simulink model "model_fuzzy"  (R2022b)
settings: Solver=VariableStepAuto  StartTime=0.0  StopTime=1000  MinStep=1e-6  RelTol=1e-4
values from neighbouring files (symbols this model uses):
  atau_D = alpha*tau_D    (= 0.455)    [FIS_script.m]    (also in PID_paramaters.m)
  tau_D = 3.64    [FIS_script.m]    (also in PID_paramaters.m)
libraries: fuzblock x2, slpidlib x1
settings Model: Creator=thapl  LastModifiedBy=thapl
settings DataIOCC: SaveFormat=Array

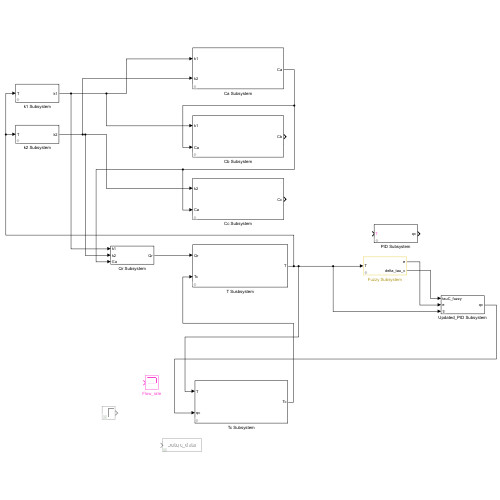
[thumbnail: Simulink's stored preview of the top-level diagram]
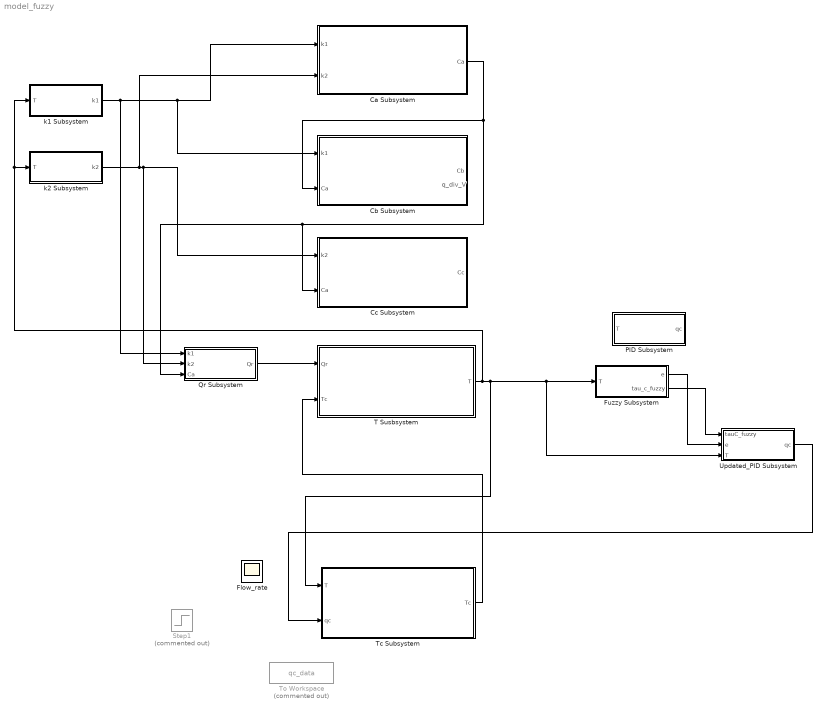
== system model_fuzzy ==
  note: q_div_V
  Ca Subsystem : Subsystem  mask{q=0.015, V=0.23, Caf=4.22}
      mask prompts: q "Feed flow rate(q)"; V "Reactor Volume(V)"; Caf "Feed Conc (Caf)"
  Cb Subsystem : Subsystem  mask{q=0.015, V=0.23, Cbf=0}
      mask prompts: q "Feed flow rate(q)"; V "Reactor Volume(V)"; Cbf "Feed Conc (Cbf)"
  Cc Subsystem : Subsystem  mask{q=0.015, V=0.23, Ccf=0}
      mask prompts: q "Feed flow rate(q)"; V "Reactor Volume(V)"; Ccf "Feed Conc (Ccf)"
  Flow_rate : Scope
  Fuzzy Subsystem : Subsystem  mask{Tset=315}
      mask prompts: Tset "Setpoint Tempreture"
  PID Subsystem : Subsystem  mask{Tset=315}
      mask prompts: Tset "Setpoint Tempreture"
  Qr Subsystem : Subsystem  mask{V=0.23, dH1=-8.6e4, dH2=-1.82e4}
      mask prompts: V "Reactor Volume (V)"; dH1 "Enthapy of Rxn1 (dH1)"; dH2 "Enthalpy of Rxn2 (dH2)"
  Step1 : Step  Commented=on  Time=200  Before=0.005  After=0.010  SampleTime=0
  T Susbsystem : Subsystem  mask{q=0.015, V=0.23, Tf=311, A=1.51, u=42.8, rho=1020, Cp=4.02}
      mask prompts: q "Reactor Flow rate (q)"; V "Reactor Volume (V)"; Tf "Inlet Fluid Temp (Tf)"; A "Contact Area (A)"; u "HTC (u)"; rho "Fluid Density (rho)"; Cp "Specific Heat capactiy (Cp)"
  Tc Subsystem : Subsystem  mask{Vc=0.21, Tcf=292, A=1.51, u=42.8, Cpc=4.182, rhoc=998}
      mask prompts: Vc "Jacket Volume (Vc)"; Tcf "Inlet Cooling Fluid Tempreture (Tcf)"; A "Contact Area (A)"; u "HTC"; Cpc "Specidic Heat Capacity of cooling fluid (Cpc)"; rhoc "Cooling Fluid Density (rhoc)"
  To Workspace : ToWorkspace  Commented=on  VariableName=qc_data  SampleTime=-1
  Updated_PID Subsystem : Subsystem  mask{t0=7.27, Kp=-480.505, tauP=27.27}
      mask prompts: t0 "Dead time"; Kp "Process Gain"; tauP "Time constant"
  k1 Subsystem : Subsystem  mask{R=8.314, k10=1.55e11, Ea1=9850*8.314}
      mask prompts: R "Universal Gas Constant(R)"; k10 "Pre exponential factor(k10)"; Ea1 "Actvation Energy(Ea1)"
  k2 Subsystem : Subsystem  mask{R=8.314, k20=4.55e25, Ea2=22019*8.314}
      mask prompts: R "Universal Gas Constant(R)"; k20 "Pre exponential factor(k10)"; Ea2 "Actvation Energy(Ea1)"
  wires:
  k1 Subsystem/1(k1) -> Ca Subsystem/1(k1), Cb Subsystem/1(k1), Qr Subsystem/1(k1)
  k2 Subsystem/1(k2) -> Qr Subsystem/2(k2), Cc Subsystem/1(k2), Ca Subsystem/2(k2)
  Ca Subsystem/1(Ca) -> Qr Subsystem/3(Ca), Cc Subsystem/2(Ca), Cb Subsystem/2(Ca)
  Tc Subsystem/1(Tc) -> T Susbsystem/2(Tc)
  T Susbsystem/1(T) -> k2 Subsystem/1(T), k1 Subsystem/1(T), Updated_PID Subsystem/3(T), Fuzzy Subsystem/1(T), Tc Subsystem/1(T)
  Qr Subsystem/1(Qr) -> T Susbsystem/1(Qr)
  Fuzzy Subsystem/1(e) -> Updated_PID Subsystem/2(e)
  Updated_PID Subsystem/1(qc) -> Tc Subsystem/2(qc)
  Fuzzy Subsystem/2(tau_c_fuzzy) -> Updated_PID Subsystem/1(tauC_fuzzy)

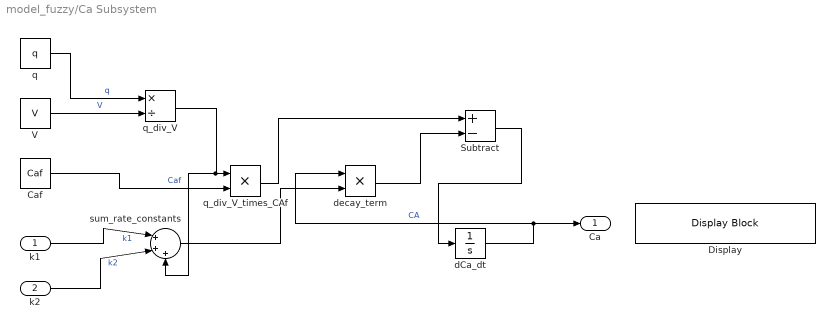
== system model_fuzzy/Ca Subsystem ==
  k1 : Inport
  k2 : Inport  Port=2
  Caf : Constant  Value=Caf
  Display : DisplayBlock  LabelPosition=Hide  Transparency=1
  Subtract : Sum  Inputs=+-
  V : Constant  Value=V
  dCa_dt : Integrator  InitialCondition=4.22
  decay_term : Product
  q : Constant  Value=q
  q_div_V : Product  Inputs=*/
  q_div_V_times_CAf : Product
  sum_rate_constants : Sum  Inputs=|+++
  Ca : Outport
  wires:
  q/1 -> q_div_V/1  "q"
  V/1 -> q_div_V/2  "V"
  q_div_V/1 -> sum_rate_constants/3, q_div_V_times_CAf/1
  Caf/1 -> q_div_V_times_CAf/2  "Caf"
  k1/1 -> sum_rate_constants/1  "k1"
  k2/1 -> sum_rate_constants/2  "k2"
  sum_rate_constants/1 -> decay_term/2
  dCa_dt/1 -> decay_term/1, Ca/1  "CA"
  decay_term/1 -> Subtract/2
  Subtract/1 -> dCa_dt/1
  q_div_V_times_CAf/1 -> Subtract/1

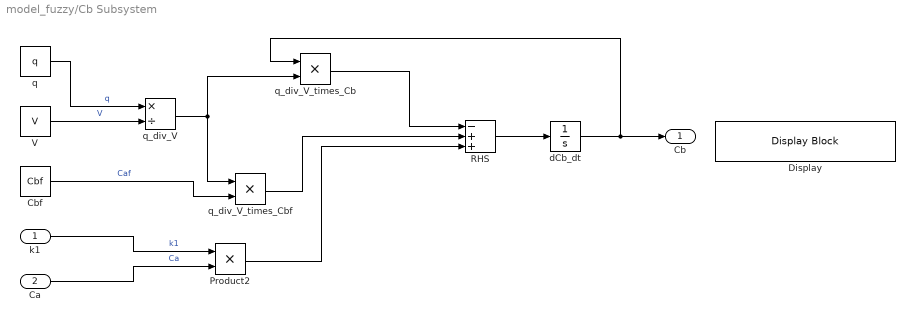
== system model_fuzzy/Cb Subsystem ==
  k1 : Inport
  Ca : Inport  Port=2
  Cbf : Constant  Value=Cbf
  Display : DisplayBlock  LabelPosition=Hide  Transparency=1
  Product2 : Product
  RHS : Sum  Inputs=-++
  V : Constant  Value=V
  dCb_dt : Integrator
  q : Constant  Value=q
  q_div_V : Product  Inputs=*/
  q_div_V_times_Cb : Product
  q_div_V_times_Cbf : Product
  Cb : Outport
  wires:
  q/1 -> q_div_V/1  "q"
  V/1 -> q_div_V/2  "V"
  q_div_V/1 -> q_div_V_times_Cb/2, q_div_V_times_Cbf/1
  Cbf/1 -> q_div_V_times_Cbf/2  "Caf"
  k1/1 -> Product2/1  "k1"
  dCb_dt/1 -> Cb/1, q_div_V_times_Cb/1
  RHS/1 -> dCb_dt/1
  Ca/1 -> Product2/2  "Ca"
  q_div_V_times_Cb/1 -> RHS/1
  q_div_V_times_Cbf/1 -> RHS/2
  Product2/1 -> RHS/3

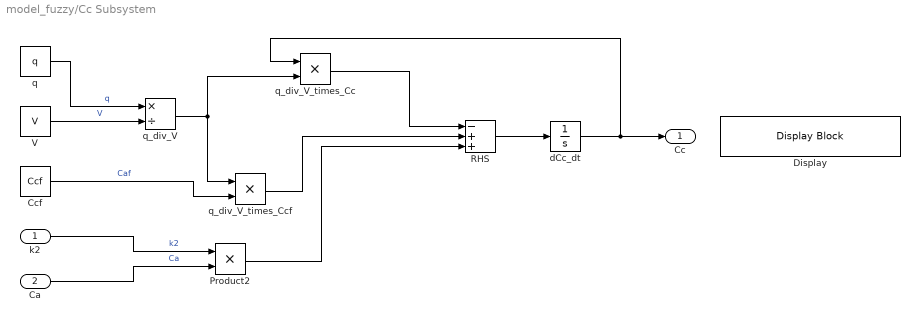
== system model_fuzzy/Cc Subsystem ==
  k2 : Inport
  Ca : Inport  Port=2
  Ccf : Constant  Value=Ccf
  Display : DisplayBlock  LabelPosition=Hide  Transparency=1
  Product2 : Product
  RHS : Sum  Inputs=-++
  V : Constant  Value=V
  dCc_dt : Integrator
  q : Constant  Value=q
  q_div_V : Product  Inputs=*/
  q_div_V_times_Cc : Product
  q_div_V_times_Ccf : Product
  Cc : Outport
  wires:
  q/1 -> q_div_V/1  "q"
  V/1 -> q_div_V/2  "V"
  q_div_V/1 -> q_div_V_times_Cc/2, q_div_V_times_Ccf/1
  Ccf/1 -> q_div_V_times_Ccf/2  "Caf"
  k2/1 -> Product2/1  "k2"
  dCc_dt/1 -> Cc/1, q_div_V_times_Cc/1
  RHS/1 -> dCc_dt/1
  Ca/1 -> Product2/2  "Ca"
  q_div_V_times_Cc/1 -> RHS/1
  q_div_V_times_Ccf/1 -> RHS/2
  Product2/1 -> RHS/3

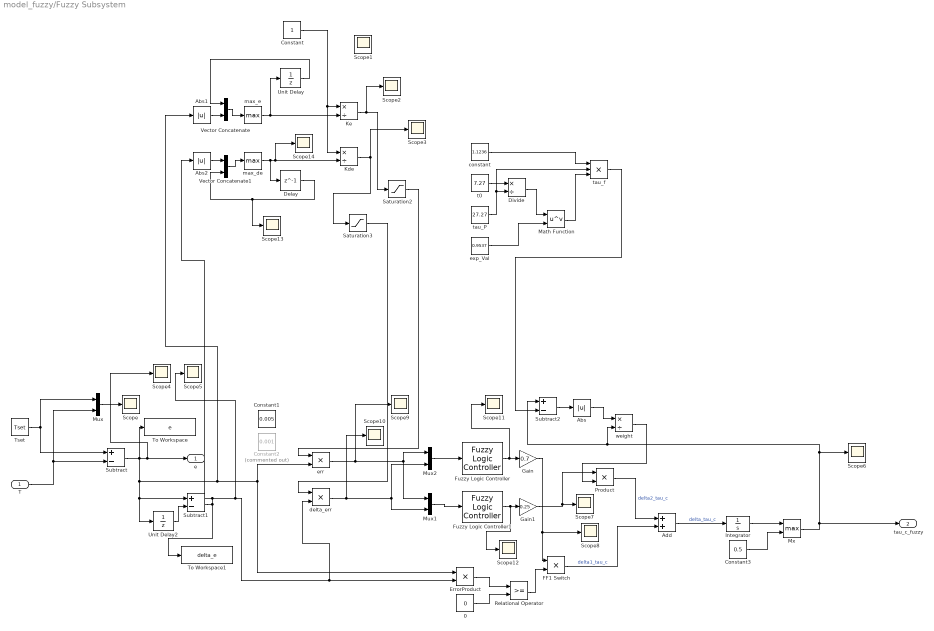
== system model_fuzzy/Fuzzy Subsystem ==
  T : Inport
  0 : Constant  Value=0
  Abs : Abs  SaturateOnIntegerOverflow=off
  Abs1 : Abs  SaturateOnIntegerOverflow=off
  Abs2 : Abs  SaturateOnIntegerOverflow=off
  Add : Sum
  Constant : Constant
  Constant1 : Constant  Value=0.005
  Constant2 : Constant  Commented=on  Value=0.001
  Constant3 : Constant  Value=0.5
  Delay : Delay  DelayLength=1  InitialCondition=0
  Divide : Product  Inputs=*/
  ErrorProduct : Product
  FF1 Switch : Product
  Fuzzy Logic Controller : fuzblock/Fuzzy Logic  Controller  FIS='FF1'  OutputSampleNumber=101  DataType=double  FuzzifiedInputs=off  RuleFiringStrengths=off  RuleOutputs=off  AggregatedOutputs=off  SimulateUsing=Interpreted execution  OutOfRangeInputValueMessage=warning  NoRuleFiredMessage=warning  EmptyOutputFuzzySetMessage=warning
  Fuzzy Logic Controller1 : fuzblock/Fuzzy Logic  Controller  FIS='FF2'  OutputSampleNumber=101  DataType=double  FuzzifiedInputs=off  RuleFiringStrengths=off  RuleOutputs=off  AggregatedOutputs=off  SimulateUsing=Interpreted execution  OutOfRangeInputValueMessage=warning  NoRuleFiredMessage=warning  EmptyOutputFuzzySetMessage=warning
  Gain : Gain  Gain=0.7
  Gain1 : Gain  Gain=0.25
  Integrator : Integrator  InitialCondition=8.6842
  Kde : Product  Inputs=*/
  Ke : Product  Inputs=*/
  Math Function : Math  Operator=pow
  Mux : Mux  Inputs=2
  Mux1 : Mux  Inputs=2
  Mux2 : Mux  Inputs=2
  Mx : MinMax  Function=max  Inputs=2
  Product : Product
  Relational Operator : RelationalOperator  OutDataTypeStr=boolean  RndMeth=Simplest  InputSameDT=off
  Saturation2 : Saturate  UpperLimit=1  LowerLimit=0.01
  Saturation3 : Saturate  UpperLimit=1  LowerLimit=0.01
  Scope{,1..14} (15 alike) : Scope
  Subtract : Sum  Inputs=+-
  Subtract1 : Sum  Inputs=+-
  Subtract2 : Sum  Inputs=+-
  To Workspace : ToWorkspace  VariableName=e  SampleTime=-1
  To Workspace1 : ToWorkspace  VariableName=delta_e  SampleTime=-1
  Tset : Constant  Value=Tset  VectorParams1D=off
  Unit Delay : UnitDelay  InitialCondition=0.1  SampleTime=-1  HasFrameUpgradeWarning=on
  Unit Delay2 : UnitDelay  InitialCondition=4  SampleTime=-1  HasFrameUpgradeWarning=on
  Vector Concatenate : Concatenate
  Vector Concatenate1 : Concatenate
  constant : Constant  Value=1.1236
  delta_err : Product
  err : Product
  exp_Val : Constant  Value=0.9537
  max_de : MinMax  Function=max
  max_e : MinMax  Function=max
  t0 : Constant  Value=7.27
  tau_P : Constant  Value=27.27
  tau_f : Product  Inputs=3
  weight : Product  Inputs=*/
  e : Outport
  tau_c_fuzzy : Outport  Port=2
  wires:
  Tset/1 -> Subtract/1, Mux/1
  Mux/1 -> Scope/1
  T/1 -> Mux/2, Subtract/2
  Unit Delay2/1 -> Subtract1/2
  Subtract2/1 -> Abs/1
  Relational Operator/1 -> FF1 Switch/2
  Subtract1/1 -> Abs2/1, Scope5/1, delta_err/2, ErrorProduct/2, To Workspace1/1
  Subtract/1 -> Unit Delay2/1, Subtract1/1, err/2, ErrorProduct/1, Abs1/1, To Workspace/1, Scope4/1, e/1
  weight/1 -> Product/2
  ErrorProduct/1 -> Relational Operator/1
  Abs/1 -> weight/1
  0/1 -> Relational Operator/2
  t0/1 -> Divide/1
  tau_P/1 -> Divide/2, tau_f/2
  Divide/1 -> Math Function/1
  exp_Val/1 -> Math Function/2
  constant/1 -> tau_f/1
  Math Function/1 -> tau_f/3
  tau_f/1 -> Subtract2/2
  FF1 Switch/1 -> Add/2  "delta1_tau_c"
  Product/1 -> Add/1  "delta2_tau_c"
  Add/1 -> Integrator/1  "delta_tau_c"
  Mux2/1 -> Fuzzy Logic Controller/1
  Mux1/1 -> Fuzzy Logic Controller1/1
  Fuzzy Logic Controller/1 -> Scope11/1, Gain/1
  Fuzzy Logic Controller1/1 -> Scope12/1, Gain1/1
  Gain/1 -> FF1 Switch/1, Scope8/1
  Gain1/1 -> Scope7/1, Product/1
  max_e/1 -> Ke/2, Unit Delay/1
  Abs1/1 -> Vector Concatenate/2
  Vector Concatenate/1 -> max_e/1
  Unit Delay/1 -> Vector Concatenate/1
  Abs2/1 -> Vector Concatenate1/1
  Vector Concatenate1/1 -> max_de/1
  Delay/1 -> Scope13/1, Vector Concatenate1/2
  max_de/1 -> Delay/1, Scope14/1, Kde/2
  Constant/1 -> Kde/1, Ke/1
  Ke/1 -> Scope2/1, Saturation2/1
  Kde/1 -> Scope3/1, Saturation3/1
  err/1 -> Scope9/1, Mux2/1, Mux1/1
  Integrator/1 -> Mx/1
  delta_err/1 -> Scope10/1, Mux1/2, Mux2/2
  Mx/1 -> tau_c_fuzzy/1, weight/2, Subtract2/1, Scope6/1
  Constant3/1 -> Mx/2
  Saturation2/1 -> err/1
  Saturation3/1 -> delta_err/1

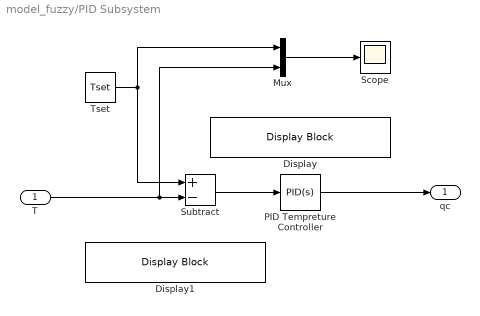
== system model_fuzzy/PID Subsystem ==
  T : Inport
  Display : DisplayBlock  LabelPosition=Hide  Transparency=1
  Display1 : DisplayBlock  LabelPosition=Hide  Transparency=1
  Mux : Mux  Inputs=2
  PID Tempreture Controller : slpidlib/PID Controller  Controller=PID  Form=Parallel  TimeDomain=Continuous-time  UseExternalTs=off  SampleTime=-1  IntegratorMethod=Forward Euler  FilterMethod=Forward Euler  ControllerParametersSource=internal  P=-0.001643  I=-0.000060  UseKiTs=off  D=-0.005975  N=100  UseFilter=on  TunerSelectOption=Transfer Function Based (PID Tuner App)  InitialConditionSource=internal  InitialConditionForIntegrator=0  InitialConditionForFilter=0  DifferentiatorICPrevScaledInput=0  ExternalReset=none  TrackingMode=off  Kt=1  LimitOutput=off  SatLimitsSource=internal  UpperSaturationLimit=inf  LowerSaturationLimit=-inf  LinearizeAsGain=on  AntiWindupMode=none  Kb=1  LimitIntegrator=off  UpperIntegratorSaturationLimit=inf  LowerIntegratorSaturationLimit=-inf  POutMin=[]  POutMax=[]  IOutMin=[]  IOutMax=[]  DOutMin=[]  DOutMax=[]  NOutMin=[]  NOutMax=[]  SumOutMin=[]  SumOutMax=[]  SaturationOutMin=[]  SaturationOutMax=[]  PParamMin=[]  PParamMax=[]  IParamMin=[]  IParamMax=[]  DParamMin=[]  DParamMax=[]  NParamMin=[]  NParamMax=[]  KbParamMin=[]  KbParamMax=[]  KtParamMin=[]  KtParamMax=[]  KbOutMin=[]  KbOutMax=[]  KtOutMin=[]  KtOutMax=[]  IntegratorOutMin=[]  IntegratorOutMax=[]  FilterOutMin=[]  FilterOutMax=[]  SumI1OutMin=[]  SumI1OutMax=[]  SumI2OutMin=[]  SumI2OutMax=[]  SumI3OutMin=[]  SumI3OutMax=[]  SumI4OutMin=[]  SumI4OutMax=[]  SumDOutMin=[]  SumDOutMax=[]  DifferentiatorOutMin=[]  DifferentiatorOutMax=[]  FilterDiffOutCoefMin=[]  FilterDiffOutCoefMax=[]  ReciprocalOutMin=[]  ReciprocalOutMax=[]  SumDenOutMin=[]  SumDenOutMax=[]  SumNumOutMin=[]  SumNumOutMax=[]  DivideOutMin=[]  DivideOutMax=[]  UdiffTsProdOutMin=[]  UdiffTsProdOutMax=[]  NTsProdOutMin=[]  NTsProdOutMax=[]  UintegralTsProdOutMin=[]  UintegralTsProdOutMax=[]  UngainTsProdOutMin=[]  UngainTsProdOutMax=[]  ClampingZeroOutDataTypeStr=Inherit: Inherit via back propagation  ClampingZeroOutMin=[]  ClampingZeroOutMax=[]  FilterDenConstantOutDataTypeStr=Inherit: Inherit via back propagation  FilterDenConstantOutMin=[]  FilterDenConstantOutMax=[]  PCopyOutDataTypeStr=Inherit: Inherit via back propagation  PCopyOutMin=[]  PCopyOutMax=[]  NCopyOutDataTypeStr=Inherit: Inherit via back propagation  NCopyOutMin=[]  NCopyOutMax=[]  IntegratorContinuousStateAttributes=''  IntegratorStateMustResolveToSignalObject=off  IntegratorRTWStateStorageClass=Auto  FilterContinuousStateAttributes=''  FilterStateMustResolveToSignalObject=off  FilterRTWStateStorageClass=Auto  ParallelPVariant=InternalParameters  IdealPVariant=Disabled  IVariant=InternalParameters  DVariant=InternalParameters  IntegratorVariant=Continuous  SatVariant=Disabled  AWVariant=Passthrough  PCopyVariant=Disabled  TRVariant=Disabled  FdbkBlocksVariant=Forward  IdealPFdbkVariant=Disabled  SatFdbkVariant=Disabled  DerivativeFilterVariant=ContFilter  NVariant=InternalParameters  NCopyVariant=Disabled  FilterICVariant=InternalICsFilter  IntegratorICVariant=InternalICs  ExternalResetVariant=Disabled  TRSumVariant=Passthrough  SumFdbkVariant=Disabled  SumVariant=Sum_PID  TsampFilterVariant=InternalTs  TsampNgainVariant=Passthrough  TsampIntegralVariant=Passthrough  ExternalSaturationOutDataTypeStr=Inherit: Same as second input
  Scope : Scope
  Subtract : Sum  Inputs=+-
  Tset : Constant  Value=Tset
  qc : Outport
  wires:
  Tset/1 -> Mux/1, Subtract/1
  Subtract/1 -> PID Tempreture Controller/1
  Mux/1 -> Scope/1
  T/1 -> Mux/2, Subtract/2
  PID Tempreture Controller/1 -> qc/1

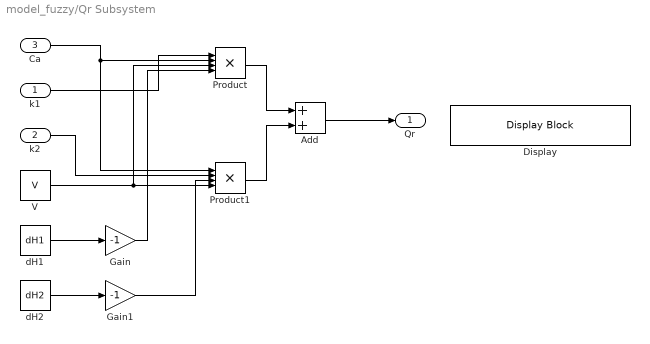
== system model_fuzzy/Qr Subsystem ==
  k1 : Inport
  k2 : Inport  Port=2
  Ca : Inport  Port=3
  Add : Sum
  Display : DisplayBlock  LabelPosition=Hide  Transparency=1
  Gain : Gain  Gain=-1
  Gain1 : Gain  Gain=-1
  Product : Product  Inputs=4
  Product1 : Product  Inputs=4
  V : Constant  Value=V
  dH1 : Constant  Value=dH1
  dH2 : Constant  Value=dH2
  Qr : Outport
  wires:
  dH1/1 -> Gain/1
  dH2/1 -> Gain1/1
  k1/1 -> Product/1
  V/1 -> Product1/4, Product/3
  Gain/1 -> Product/4
  Ca/1 -> Product1/1, Product/2
  k2/1 -> Product1/2
  Gain1/1 -> Product1/3
  Product/1 -> Add/1
  Product1/1 -> Add/2
  Add/1 -> Qr/1

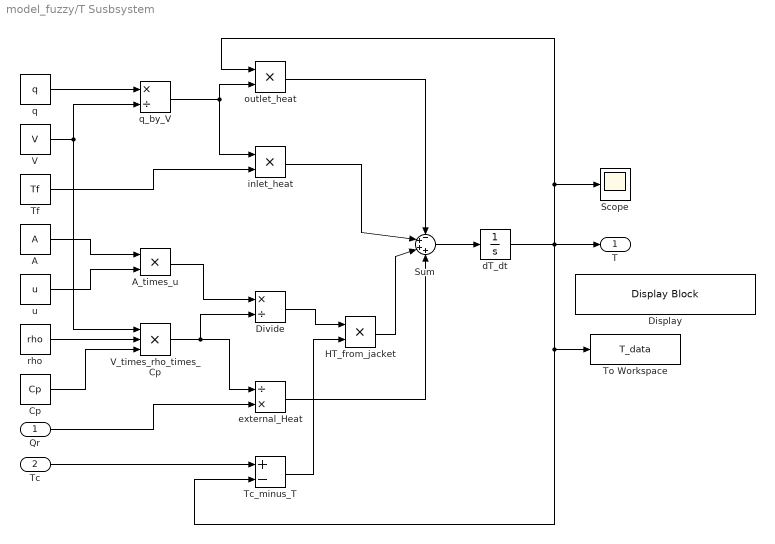
== system model_fuzzy/T Susbsystem ==
  Qr : Inport
  Tc : Inport  Port=2
  A : Constant  Value=A
  A_times_u : Product
  Cp : Constant  Value=Cp
  Display : DisplayBlock  LabelPosition=Hide  Transparency=1
  Divide : Product  Inputs=*/
  HT_from_jacket : Product
  Scope : Scope
  Sum : Sum  Inputs=-+++
  Tc_minus_T : Sum  Inputs=+-
  Tf : Constant  Value=Tf
  To Workspace : ToWorkspace  VariableName=T_data  SampleTime=-1
  V : Constant  Value=V
  V_times_rho_times_Cp : Product  Inputs=3
  dT_dt : Integrator  InitialCondition=310
  external_Heat : Product  Inputs=/*
  inlet_heat : Product
  outlet_heat : Product
  q : Constant  Value=q
  q_by_V : Product  Inputs=*/
  rho : Constant  Value=rho
  u : Constant  Value=u
  T : Outport
  wires:
  q/1 -> q_by_V/1
  V/1 -> V_times_rho_times_Cp/1, q_by_V/2
  q_by_V/1 -> outlet_heat/2, inlet_heat/1
  Tf/1 -> inlet_heat/2
  A/1 -> A_times_u/1
  u/1 -> A_times_u/2
  rho/1 -> V_times_rho_times_Cp/2
  Cp/1 -> V_times_rho_times_Cp/3
  A_times_u/1 -> Divide/1
  V_times_rho_times_Cp/1 -> external_Heat/1, Divide/2
  Divide/1 -> HT_from_jacket/1
  Tc_minus_T/1 -> HT_from_jacket/2
  Qr/1 -> external_Heat/2
  outlet_heat/1 -> Sum/1
  inlet_heat/1 -> Sum/2
  HT_from_jacket/1 -> Sum/3
  external_Heat/1 -> Sum/4
  Sum/1 -> dT_dt/1
  dT_dt/1 -> Scope/1, outlet_heat/1, T/1, To Workspace/1, Tc_minus_T/2
  Tc/1 -> Tc_minus_T/1

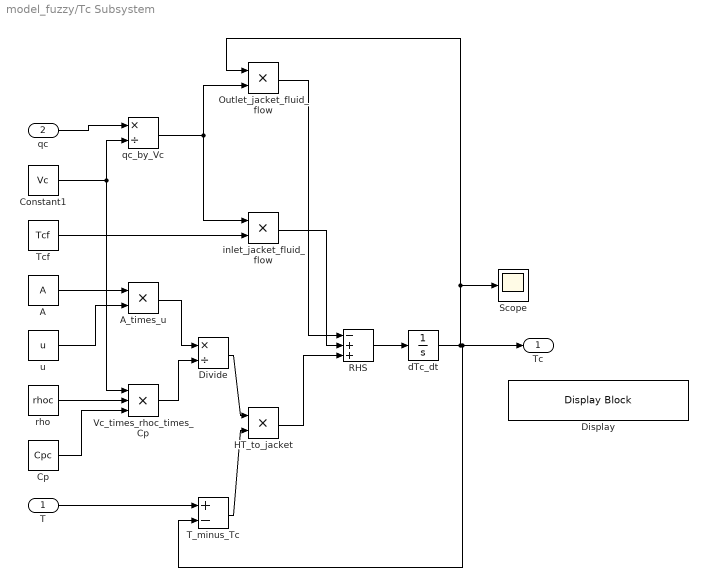
== system model_fuzzy/Tc Subsystem ==
  T : Inport
  qc : Inport  Port=2
  A : Constant  Value=A
  A_times_u : Product
  Constant1 : Constant  Value=Vc
  Cp : Constant  Value=Cpc
  Display : DisplayBlock  LabelPosition=Hide  Transparency=1
  Divide : Product  Inputs=*/
  HT_to_jacket : Product
  Outlet_jacket_fluid_flow : Product
  RHS : Sum  Inputs=-++
  Scope : Scope
  T_minus_Tc : Sum  Inputs=+-
  Tcf : Constant  Value=Tcf
  Vc_times_rhoc_times_Cp : Product  Inputs=3
  dTc_dt : Integrator  InitialCondition=290
  inlet_jacket_fluid_flow : Product
  qc_by_Vc : Product  Inputs=*/
  rho : Constant  Value=rhoc
  u : Constant  Value=u
  Tc : Outport
  wires:
  qc/1 -> qc_by_Vc/1
  Constant1/1 -> Vc_times_rhoc_times_Cp/1, qc_by_Vc/2
  qc_by_Vc/1 -> Outlet_jacket_fluid_flow/2, inlet_jacket_fluid_flow/1
  Tcf/1 -> inlet_jacket_fluid_flow/2
  A/1 -> A_times_u/1
  u/1 -> A_times_u/2
  rho/1 -> Vc_times_rhoc_times_Cp/2
  Cp/1 -> Vc_times_rhoc_times_Cp/3
  A_times_u/1 -> Divide/1
  Vc_times_rhoc_times_Cp/1 -> Divide/2
  T/1 -> T_minus_Tc/1
  Divide/1 -> HT_to_jacket/1
  T_minus_Tc/1 -> HT_to_jacket/2
  HT_to_jacket/1 -> RHS/3
  inlet_jacket_fluid_flow/1 -> RHS/2
  RHS/1 -> dTc_dt/1
  dTc_dt/1 -> Scope/1, Outlet_jacket_fluid_flow/1, Tc/1, T_minus_Tc/2
  Outlet_jacket_fluid_flow/1 -> RHS/1

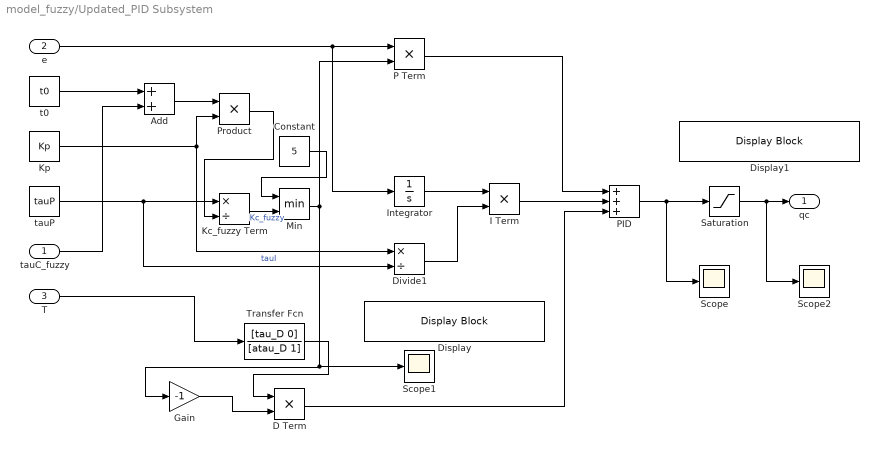
== system model_fuzzy/Updated_PID Subsystem ==
  tauC_fuzzy : Inport
  e : Inport  Port=2
  T : Inport  Port=3
  Add : Sum
  Constant : Constant  Value=5
  D Term : Product
  Display : DisplayBlock  LabelPosition=Hide  Transparency=1
  Display1 : DisplayBlock  LabelPosition=Hide  Transparency=1
  Divide1 : Product  Inputs=*/
  Gain : Gain  Gain=-1
  I Term : Product
  Integrator : Integrator
  Kc_fuzzy Term : Product  Inputs=*/
  Kp : Constant  Value=Kp
  Min : MinMax  Inputs=2
  P Term : Product
  PID : Sum  Inputs=+++
  Product : Product
  Saturation : Saturate  UpperLimit=0.015  LowerLimit=0
  Scope : Scope
  Scope1 : Scope
  Scope2 : Scope
  Transfer Fcn : TransferFcn  Numerator=[tau_D 0]  Denominator=[atau_D 1]  ParameterTunability=Optimized
  t0 : Constant  Value=t0
  tauP : Constant  Value=tauP
  qc : Outport
  wires:
  t0/1 -> Add/1
  tauC_fuzzy/1 -> Add/2
  Add/1 -> Product/1
  Kp/1 -> Divide1/1, Product/2
  tauP/1 -> Divide1/2, Kc_fuzzy Term/1  "tauI"
  Product/1 -> Kc_fuzzy Term/2
  e/1 -> Integrator/1, P Term/1
  Integrator/1 -> I Term/1
  Divide1/1 -> I Term/2
  T/1 -> Transfer Fcn/1
  Gain/1 -> D Term/2
  Transfer Fcn/1 -> D Term/1
  P Term/1 -> PID/1
  I Term/1 -> PID/2
  D Term/1 -> PID/3
  PID/1 -> Saturation/1, Scope/1
  Saturation/1 -> Scope2/1, qc/1
  Kc_fuzzy Term/1 -> Min/2  "Kc_fuzzy"
  Min/1 -> P Term/2, Gain/1, Scope1/1
  Constant/1 -> Min/1

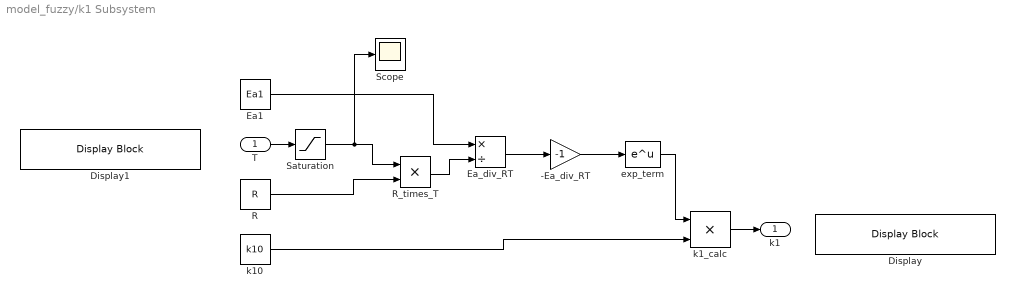
== system model_fuzzy/k1 Subsystem ==
  T : Inport
  -Ea_div_RT : Gain  Gain=-1
  Display : DisplayBlock  LabelPosition=Hide  Transparency=1
  Display1 : DisplayBlock  LabelPosition=Hide  Transparency=1
  Ea1 : Constant  Value=Ea1
  Ea_div_RT : Product  Inputs=*/
  R : Constant  Value=R
  R_times_T : Product
  Saturation : Saturate  UpperLimit=Inf  LowerLimit=0.001
  Scope : Scope
  exp_term : Math
  k10 : Constant  Value=k10
  k1_calc : Product
  k1 : Outport
  wires:
  R/1 -> R_times_T/2
  Ea1/1 -> Ea_div_RT/1
  R_times_T/1 -> Ea_div_RT/2
  k10/1 -> k1_calc/2
  k1_calc/1 -> k1/1
  Ea_div_RT/1 -> -Ea_div_RT/1
  -Ea_div_RT/1 -> exp_term/1
  exp_term/1 -> k1_calc/1
  T/1 -> Saturation/1
  Saturation/1 -> Scope/1, R_times_T/1

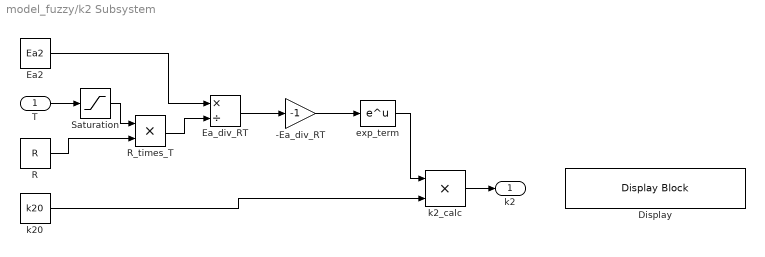
== system model_fuzzy/k2 Subsystem ==
  T : Inport
  -Ea_div_RT : Gain  Gain=-1
  Display : DisplayBlock  LabelPosition=Hide  Transparency=1
  Ea2 : Constant  Value=Ea2
  Ea_div_RT : Product  Inputs=*/
  R : Constant  Value=R
  R_times_T : Product
  Saturation : Saturate  UpperLimit=Inf  LowerLimit=0.001
  exp_term : Math
  k20 : Constant  Value=k20
  k2_calc : Product
  k2 : Outport
  wires:
  R/1 -> R_times_T/2
  Ea2/1 -> Ea_div_RT/1
  R_times_T/1 -> Ea_div_RT/2
  k20/1 -> k2_calc/2
  k2_calc/1 -> k2/1
  Ea_div_RT/1 -> -Ea_div_RT/1
  -Ea_div_RT/1 -> exp_term/1
  exp_term/1 -> k2_calc/1
  T/1 -> Saturation/1
  Saturation/1 -> R_times_T/1
